simulink model "verify_Window_Control_mdl"  (R2016b)
settings: Solver=ode45  StartTime=0.0  StopTime=3*24*3600  MaxStep=300  RelTol=1e-3  EnableMultiTasking=on
libraries: simulink x2, carnot x1
settings Model: Creator=drhf  LastModifiedBy=drhf
settings DataIOCC: SaveFormat=Array  SignalLoggingSaveFormat=ModelDataLogs
settings OptimizationCC: ExpressionDepthLimit=2147483647  LifeSpan=inf
settings DebuggingCC: UnderspecifiedInitializationDetection=Classic  MergeDetectMultiDrivingBlocksExec=none  SolverPrmCheckMsg=warning  FcnCallInpInsideContextMsg=warning  StateNameClashWarn=warning  SFUnexpectedBacktrackingDiag=warning  SFNoUnconditionalDefaultTransitionDiag=warning  SFExecutionAtInitializationDiag=none
settings HardwareCC: ProdBitPerPointer=32  ProdBitPerSizeT=32  ProdBitPerPtrDiffT=32  ProdLargestAtomicFloat=None  ProdIntDivRoundTo=Undefined  ProdEndianess=Unspecified  ProdWordSize=32  ProdHWDeviceType=32-bit Generic
settings ModelReferenceCC: PropagateSignalLabelsOutOfModel=off
settings GRTTargetCC: TargetLangStandard=C89/C90 (ANSI)  GeneratePreprocessorConditionals=Disable all  CombineOutputUpdateFcns=off  GRTInterface=on
settings ConfigComp: CovMetricSettings=dw  CovHtmlReporting=on  CovSaveCumulativeToWorkspaceVar=on  CovSaveSingleToWorkspaceVar=on  CovExternalEMLEnable=off

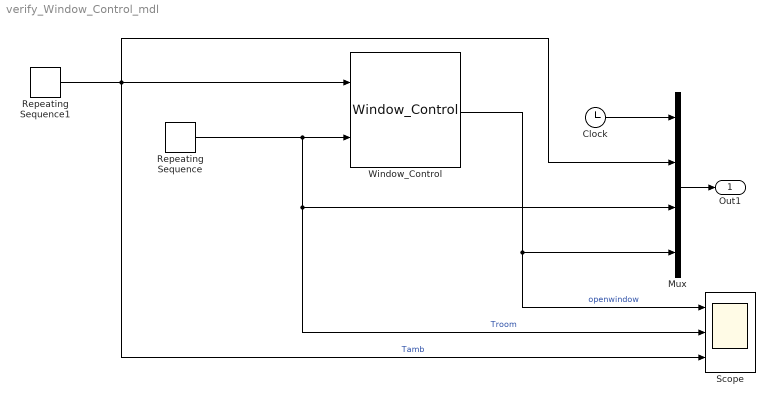
== system verify_Window_Control_mdl ==
  Clock : Clock
  Mux : Mux
  Repeating Sequence : simulink/Sources/Repeating Sequence  rep_seq_t=[ 0 10 11 13 14 18 19 23 24]*3600  rep_seq_y=[20 20 25 25 20 20 25 25 20]
  Repeating Sequence1 : simulink/Sources/Repeating Sequence  rep_seq_t=[0 24 24.1 48 48.1 72]*3600  rep_seq_y=[22 22 24 24 0 0]
  Scope : Scope  NumInputPorts=3
  Window_Control : carnot/Control/Window_Control  Topen=24  Tclose=23  TrAboveTa=2  TaTooCold=12  timeFIR=1  TaIni=12  starttime=8  stoptime=22
  Out1 : Outport
  wires:
  Window_Control/1 -> Scope/1, Mux/4  "openwindow"
  Repeating Sequence/1 -> Scope/2, Mux/3, Window_Control/2  "Troom"
  Repeating Sequence1/1 -> Scope/3, Mux/2, Window_Control/1  "Tamb"
  Clock/1 -> Mux/1
  Mux/1 -> Out1/1
